simulink subsystem "rss_MotoTempHiLvl1Dia"  (R2023a)
settings: Solver=VariableStepAuto  StartTime=0.0  StopTime=10.0  RelTol=1e-3
undefined symbols (not defined in the file): ENM_TYPE_FALT, Gu16_ctMotoTempHiLvl1ConfCnt_C, Gu16_ctMotoTempHiLvl1RcvyCnt_C, Gu8_tMotoTempHiLvl1ConfTrs_C, Gu8_tMotoTempHiLvl1RcvyTrs_C
libraries: vhit_control_library x1, lib_fault_definiteness x1
settings Model: Creator=xiaoqiang.yuan  LastModifiedBy=xiaoqiang.yuan

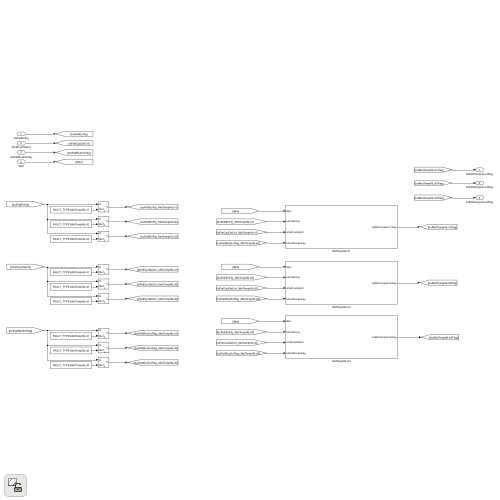
[thumbnail: Simulink's stored preview of the top-level diagram]
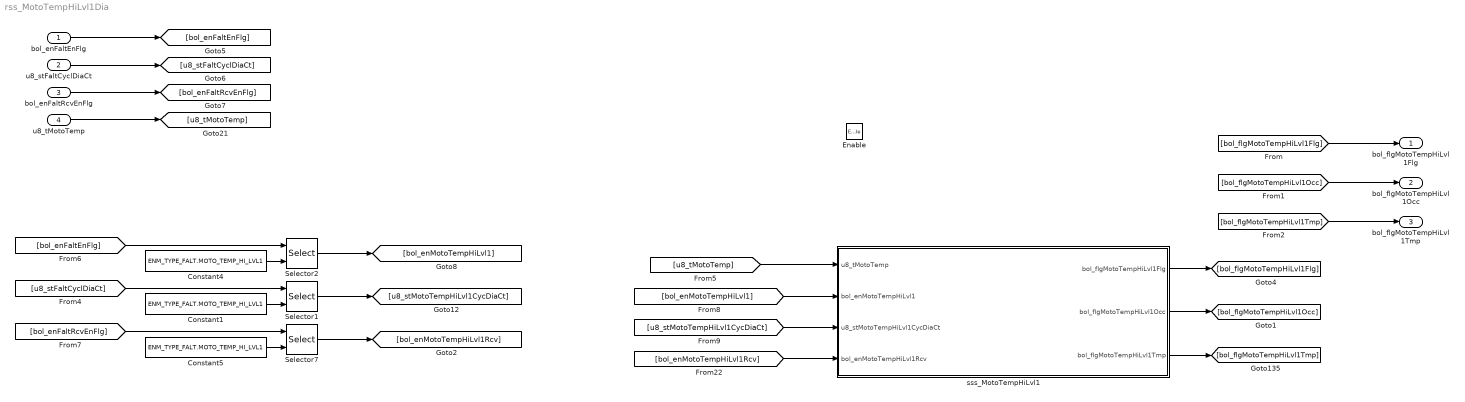
== system rss_MotoTempHiLvl1Dia ==
  bol_enFaltEnFlg : Inport  OutDataTypeStr=boolean
  u8_stFaltCyclDiaCt : Inport  Port=2  OutDataTypeStr=uint8
  bol_enFaltRcvEnFlg : Inport  Port=3  OutDataTypeStr=boolean
  u8_tMotoTemp : Inport  Port=4  OutDataTypeStr=dt_Temp_u8p0bn40
  Enable : EnablePort
  Constant1 : Constant  Value=ENM_TYPE_FALT.MOTO_TEMP_HI_LVL1
  Constant4 : Constant  Value=ENM_TYPE_FALT.MOTO_TEMP_HI_LVL1
  Constant5 : Constant  Value=ENM_TYPE_FALT.MOTO_TEMP_HI_LVL1
  Selector1 : Selector  IndexMode=Zero-based  InputPortWidth=Cdbl_numFaltDiaNum  IndexOptions=Index vector (port)  Indices=[1 3]  OutputSizes=1
  Selector2 : Selector  IndexMode=Zero-based  InputPortWidth=Cdbl_numFaltDiaNum  IndexOptions=Index vector (port)  Indices=[1 3]  OutputSizes=1
  Selector7 : Selector  IndexMode=Zero-based  InputPortWidth=Cdbl_numFaltDiaNum  IndexOptions=Index vector (port)  Indices=[1 3]  OutputSizes=1
  sss_MotoTempHiLvl1 : Subsystem
  bol_flgMotoTempHiLvl1Flg : Outport  OutDataTypeStr=boolean
  bol_flgMotoTempHiLvl1Occ : Outport  Port=2  OutDataTypeStr=boolean
  bol_flgMotoTempHiLvl1Tmp : Outport  Port=3  OutDataTypeStr=boolean
  wires:
  [bol_flgMotoTempHiLvl1Occ] -> bol_flgMotoTempHiLvl1Occ/1
  [bol_flgMotoTempHiLvl1Flg] -> bol_flgMotoTempHiLvl1Flg/1
  Selector2/1 -> [bol_enMotoTempHiLvl1]
  [bol_enMotoTempHiLvl1Rcv] -> sss_MotoTempHiLvl1/4(bol_enMotoTempHiLvl1Rcv)
  Selector7/1 -> [bol_enMotoTempHiLvl1Rcv]
  [bol_enFaltRcvEnFlg] -> Selector7/1
  Constant4/1 -> Selector2/2
  u8_tMotoTemp/1 -> [u8_tMotoTemp]
  Selector1/1 -> [u8_stMotoTempHiLvl1CycDiaCt]
  Constant1/1 -> Selector1/2
  [u8_tMotoTemp] -> sss_MotoTempHiLvl1/1(u8_tMotoTemp)
  [bol_enMotoTempHiLvl1] -> sss_MotoTempHiLvl1/2(bol_enMotoTempHiLvl1)
  [bol_enFaltEnFlg] -> Selector2/1
  u8_stFaltCyclDiaCt/1 -> [u8_stFaltCyclDiaCt]
  bol_enFaltRcvEnFlg/1 -> [bol_enFaltRcvEnFlg]
  [u8_stFaltCyclDiaCt] -> Selector1/1
  [u8_stMotoTempHiLvl1CycDiaCt] -> sss_MotoTempHiLvl1/3(u8_stMotoTempHiLvl1CycDiaCt)
  bol_enFaltEnFlg/1 -> [bol_enFaltEnFlg]
  Constant5/1 -> Selector7/2
  sss_MotoTempHiLvl1/1(bol_flgMotoTempHiLvl1Flg) -> [bol_flgMotoTempHiLvl1Flg]
  sss_MotoTempHiLvl1/2(bol_flgMotoTempHiLvl1Occ) -> [bol_flgMotoTempHiLvl1Occ]
  [bol_flgMotoTempHiLvl1Tmp] -> bol_flgMotoTempHiLvl1Tmp/1
  sss_MotoTempHiLvl1/3(bol_flgMotoTempHiLvl1Tmp) -> [bol_flgMotoTempHiLvl1Tmp]

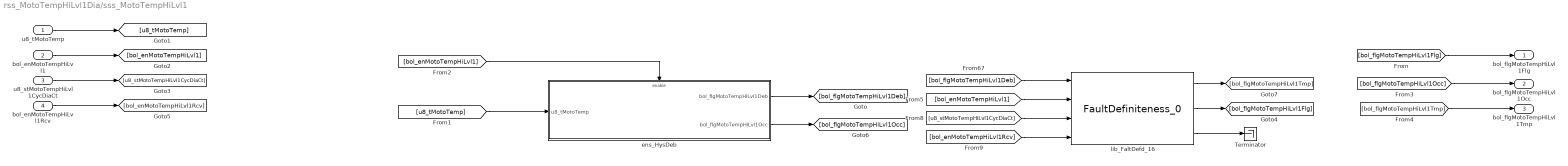
== system rss_MotoTempHiLvl1Dia/sss_MotoTempHiLvl1 ==
  u8_tMotoTemp : Inport
  bol_enMotoTempHiLvl1 : Inport  Port=2
  u8_stMotoTempHiLvl1CycDiaCt : Inport  Port=3
  bol_enMotoTempHiLvl1Rcv : Inport  Port=4
  Terminator : Terminator
  ens_HysDeb : Subsystem
  lib_FaltDefd_16 : lib_fault_definiteness/FaultDefiniteness_0  lb_FaltWaitRecvCnt=Gu16_ctMotoTempHiLvl1ConfCnt_C
  bol_flgMotoTempHiLvl1Flg : Outport
  bol_flgMotoTempHiLvl1Occ : Outport  Port=2
  bol_flgMotoTempHiLvl1Tmp : Outport  Port=3
  wires:
  [bol_flgMotoTempHiLvl1Tmp] -> bol_flgMotoTempHiLvl1Tmp/1
  [bol_flgMotoTempHiLvl1Occ] -> bol_flgMotoTempHiLvl1Occ/1
  ens_HysDeb/2(bol_flgMotoTempHiLvl1Occ) -> [bol_flgMotoTempHiLvl1Occ]
  lib_FaltDefd_16/1 -> [bol_flgMotoTempHiLvl1Tmp]
  lib_FaltDefd_16/2 -> [bol_flgMotoTempHiLvl1Flg]
  lib_FaltDefd_16/3 -> Terminator/1
  [bol_enMotoTempHiLvl1] -> ens_HysDeb/Enable
  [u8_tMotoTemp] -> ens_HysDeb/1(u8_tMotoTemp)
  ens_HysDeb/1(bol_flgMotoTempHiLvl1Deb) -> [bol_flgMotoTempHiLvl1Deb]
  bol_enMotoTempHiLvl1Rcv/1 -> [bol_enMotoTempHiLvl1Rcv]
  u8_stMotoTempHiLvl1CycDiaCt/1 -> [u8_stMotoTempHiLvl1CycDiaCt]
  bol_enMotoTempHiLvl1/1 -> [bol_enMotoTempHiLvl1]
  [bol_flgMotoTempHiLvl1Flg] -> bol_flgMotoTempHiLvl1Flg/1
  u8_tMotoTemp/1 -> [u8_tMotoTemp]
  [bol_enMotoTempHiLvl1Rcv] -> lib_FaltDefd_16/4
  [u8_stMotoTempHiLvl1CycDiaCt] -> lib_FaltDefd_16/3
  [bol_enMotoTempHiLvl1] -> lib_FaltDefd_16/2
  [bol_flgMotoTempHiLvl1Deb] -> lib_FaltDefd_16/1

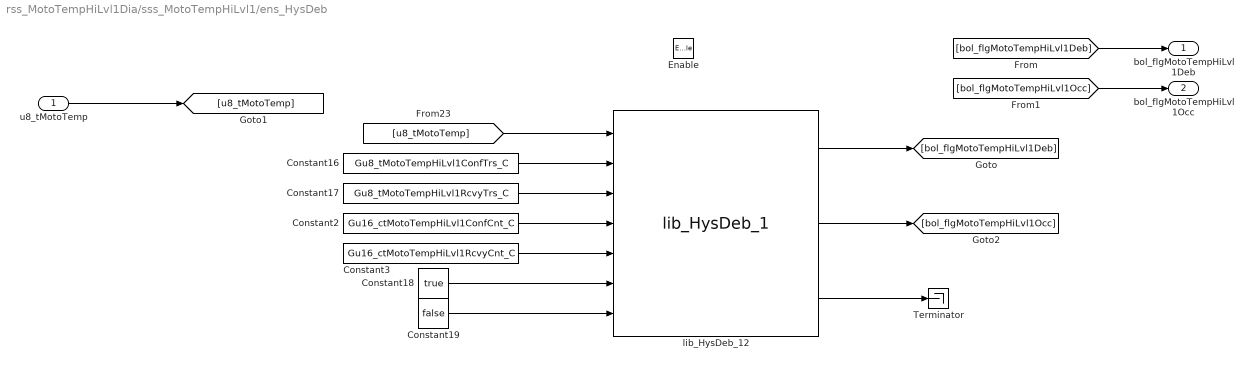
== system rss_MotoTempHiLvl1Dia/sss_MotoTempHiLvl1/ens_HysDeb ==
  u8_tMotoTemp : Inport
  Enable : EnablePort
  Constant16 : Constant  Value=Gu8_tMotoTempHiLvl1ConfTrs_C
  Constant17 : Constant  Value=Gu8_tMotoTempHiLvl1RcvyTrs_C
  Constant18 : Constant  Value=true  OutDataTypeStr=boolean
  Constant19 : Constant  Value=false  OutDataTypeStr=boolean
  Constant2 : Constant  Value=Gu16_ctMotoTempHiLvl1ConfCnt_C
  Constant3 : Constant  Value=Gu16_ctMotoTempHiLvl1RcvyCnt_C
  Terminator : Terminator
  lib_HysDeb_12 : vhit_control_library/lib_HysDeb_1  lb_parInitOutp=0
  bol_flgMotoTempHiLvl1Deb : Outport
  bol_flgMotoTempHiLvl1Occ : Outport  Port=2
  wires:
  [bol_flgMotoTempHiLvl1Occ] -> bol_flgMotoTempHiLvl1Occ/1
  lib_HysDeb_12/2 -> [bol_flgMotoTempHiLvl1Occ]
  lib_HysDeb_12/3 -> Terminator/1
  Constant3/1 -> lib_HysDeb_12/5
  Constant2/1 -> lib_HysDeb_12/4
  Constant19/1 -> lib_HysDeb_12/7
  Constant18/1 -> lib_HysDeb_12/6
  Constant17/1 -> lib_HysDeb_12/3
  Constant16/1 -> lib_HysDeb_12/2
  [u8_tMotoTemp] -> lib_HysDeb_12/1
  u8_tMotoTemp/1 -> [u8_tMotoTemp]
  [bol_flgMotoTempHiLvl1Deb] -> bol_flgMotoTempHiLvl1Deb/1
  lib_HysDeb_12/1 -> [bol_flgMotoTempHiLvl1Deb]
